simulink model "autonomous_drone"  (R2022a)
settings: Solver=FixedStepAuto  StartTime=0.0  StopTime=inf  FixedStep=sample_time  RelTol=1e-3
PostLoadFcn:
  | addpath("../");
  | load('drone_buses.mat');
InitFcn:
  | rng('shuffle');
StartFcn:
  | rng('shuffle');
model workspace (MAT data in the model file):
  SL_ROS_VariableLengthArrays_MaxSizes.CommonInfo.ArrayTruncateAction = 'EmitWarning'
  SL_ROS_VariableLengthArrays_MaxSizes.MsgTypeMap = containers.Map
  SL_ROS_VariableLengthArrays_MaxSizes.MsgTypeMap.serialization.keys = {'sensor_msgs/Image'}
  SL_ROS_VariableLengthArrays_MaxSizes.MsgTypeMap.serialization.values{1}(1).PropertyName = 'Data'
  SL_ROS_VariableLengthArrays_MaxSizes.MsgTypeMap.serialization.values{1}(1).DataType = 'uint8'
  SL_ROS_VariableLengthArrays_MaxSizes.MsgTypeMap.serialization.values{1}(1).MaxLength = 230400
  SL_ROS_VariableLengthArrays_MaxSizes.MsgTypeMap.serialization.values{1}(2).PropertyName = 'Encoding'
  SL_ROS_VariableLengthArrays_MaxSizes.MsgTypeMap.serialization.values{1}(2).DataType = 'uint8'
  SL_ROS_VariableLengthArrays_MaxSizes.MsgTypeMap.serialization.values{1}(2).MaxLength = 128
  SL_ROS_VariableLengthArrays_MaxSizes.MsgTypeMap.serialization.uniformity = 0
  SL_ROS_VariableLengthArrays_MaxSizes.MsgTypeMap.serialization.keyType = 'char'
  SL_ROS_VariableLengthArrays_MaxSizes.MsgTypeMap.serialization.valueType = 'any'
  cmd_calibration = 0.4
  sample_time = 0.05
undefined symbols (not defined in the file or in its folder): Orientation, Position
libraries: robotlib x11, simulink_extras x4, simulink x2, aerolibanimutils x1, vrlib x1
settings Model: Creator=rcasado  LastModifiedBy=usuario
settings SolverCC: AlgebraicLoopSolver=TrustRegion
settings DataIOCC: ReturnWorkspaceOutputs=off
settings OptimizationCC: EnhancedBackFolding=on  PassReuseOutputArgsAs=Individual arguments  ZeroExternalMemoryAtStartup=off  ZeroInternalMemoryAtStartup=off  MaxStackSize=64  OptimizeBlockOrder=speed  DifferentSizesBufferReuse=on  OptimizationCustomize=off  EfficientTunableParamExpr=on
settings DebuggingCC: ParameterTunabilityLossMsg=error  UnconnectedInputMsg=warning  UnconnectedOutputMsg=warning  UnconnectedLineMsg=warning  BusObjectLabelMismatch=none  PregeneratedLibrarySubsystemCodeDiagnostic=none  SFMachineParentedDataDiag=warning  ArithmeticOperatorsInVariantConditions=warning
settings HardwareCC: ProdBitPerPointer=32  ProdBitPerSizeT=32  ProdBitPerPtrDiffT=32  ProdLargestAtomicFloat=None  ProdIntDivRoundTo=Undefined  ProdEndianess=Unspecified  ProdWordSize=32  ProdHWDeviceType=Generic->Unspecified (assume 32-bit Generic)  UseEmbeddedCoderFeatures=off
settings SFSimCC: SimUseLocalCustomCode=off  MATLABDynamicMemAlloc=off  CustomCodeUndefinedFunction=UseInterfaceOnly
settings RTWCC: SystemTargetFile=ert.tlc  HardwareBoard=Robot Operating System (ROS)  TLCOptions="-aInlineSetEventsForThisBaseRateFcn=TLC_FALSE -aSuppressMultiTaskScheduler=TLC_FALSE  -aRateBasedStepFcn=0"  TemplateMakefile=ert_default_tmf  RTWUseLocalCustomCode=off  Toolchain=Catkin  TargetLang=C++  DLArmComputeVersion=19.05
settings CodeAppCC: ForceParamTrailComments=on  IgnoreCustomStorageClasses=off  OperatorAnnotations=on  SimulinkDataObjDesc=on  SFDataObjDesc=on  InsertBlockDesc=on
settings ERTTargetCC: SupportNonInlinedSFcns=on

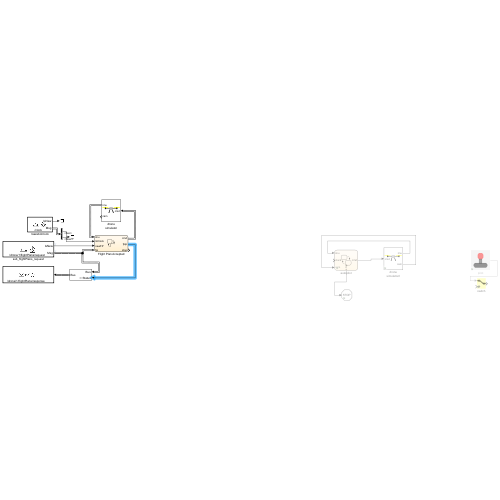
[thumbnail: Simulink's stored preview of the top-level diagram]
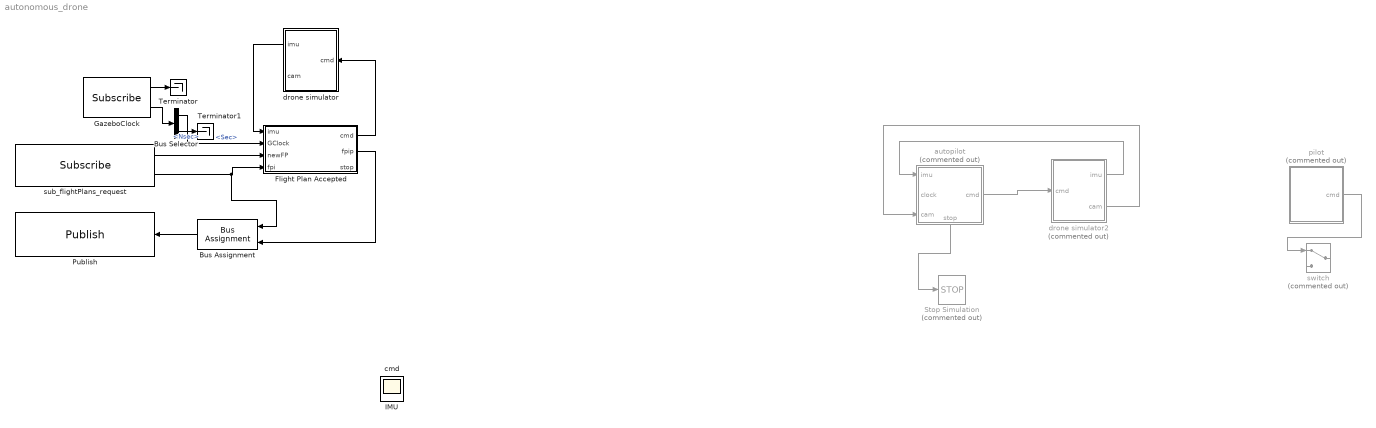
== system autonomous_drone ==
  Bus Assignment : BusAssignment  AssignedSignals=Status
  Bus Selector : BusSelector  OutputSignals=Clock_.Sec,Clock_.Nsec
  Flight Plan Accepted : Stateflow chart  TreatAsAtomicUnit=on
  GazeboClock : robotlib/Subscribe  topicSource=Specify your own  topic=/clock  messageType=rosgraph_msgs/Clock  SampleTime=-1  legacyBusStruct=off  messageQueueLength=1
  Publish : robotlib/Publish  topicSource=Specify your own  topic=/drone/1/flightPlans/response  messageType=siam_main/FlightPlan  legacyBusStruct=off  messageQueueLength=1
  Stop Simulation : Stop  Commented=on
  Terminator : Terminator
  Terminator1 : Terminator
  autopilot : Stateflow chart  Commented=on  TreatAsAtomicUnit=on
      settings: PortSchema="{\"entries\":[{\"content\":{\"sides\":[{\"content\":{\"connectorIds\":[\"In1\",\"In2\",\"In3\"]},\"type\":\"ConnectorPlacement.EquallySpacedRectSide\",\"uuid\":\"89f99594-5326-40e9-9243-02e6688f7e7f\"},{\"content\":{\"connectorIds\":[\"Out1\"],\"side\":\"RIGHT\"},\"type\":\"ConnectorPlacement.EquallySpacedRectSide\",\"uuid\":\"fb6fc64d-4bbc-4560-b28a-cb6226770084\"},{\"content\":{\"connectorIds\":[],\"side\":\"TOP\"},\"type\":\"ConnectorPlacement.EquallySpacedRectSide\",\"uuid\":\"e2b7224a-c622-478e-893e-aabf8760397b\"},{\"content\":{\"connectorIds\":[\"Out2\"],\"side\":\"BOTTOM\"},\"type\":\"ConnectorPlacement.EquallySpacedRectSide\",\"uuid\":\"7db274c0-1c25-455b-8085-b078913bfcbd\"}]},\"type\":\"ConnectorPlacement.EquallySpacedConnector\",\"uuid\":\"69f5fc45-7c88-4079-aa06-728f92b8ad33\"}],\"packageUris\":[\"http://schema.mathworks.com/mf0/Connector/R2020b\"],\"version\":\"1.0\"}"
  drone simulator : Subsystem
      mask Display:
      | patch([50 -50 -50 50], [40 40 -60 -60], [1 1 1])
      | 
      | patch([8 -8 -8 8], [6 6 -6 -6], [0.7 0.7 0.7])
      | 
      | patch([ 8  8  28  28], [2 0 0 2], [0.5 0.5 0.5])
      | patch([-8 -8 -28 -28], [2 0 0 2], [0.5 0.5 0.5])
      | 
      | patch([ 30  46  30  14], [6 5 4 5], [1 1 0])
      | patch([-30 -46 -30 -14], [6 5 4 5], [1 1 0])
      | 
      | patch([ 28  28  32  32], [4 -2 -2 4], [0 0 0])
      | patch([-28 -28 -32 -32], [4 -2 -2 4], [0 0 0])
      | 
      | patch([ 8  12  11  7], [-6 -18 -18 -6], [0 0 0])
      | patch([-8 -12 -11 -7], [-6 -18 -18 -6], [0 0 0])
  drone simulator2 : Subsystem  Commented=on
      mask Display:
      | patch([50 -50 -50 50], [40 40 -60 -60], [1 1 1])
      | 
      | patch([8 -8 -8 8], [6 6 -6 -6], [0.7 0.7 0.7])
      | 
      | patch([ 8  8  28  28], [2 0 0 2], [0.5 0.5 0.5])
      | patch([-8 -8 -28 -28], [2 0 0 2], [0.5 0.5 0.5])
      | 
      | patch([ 30  46  30  14], [6 5 4 5], [1 1 0])
      | patch([-30 -46 -30 -14], [6 5 4 5], [1 1 0])
      | 
      | patch([ 28  28  32  32], [4 -2 -2 4], [0 0 0])
      | patch([-28 -28 -32 -32], [4 -2 -2 4], [0 0 0])
      | 
      | patch([ 8  12  11  7], [-6 -18 -18 -6], [0 0 0])
      | patch([-8 -12 -11 -7], [-6 -18 -18 -6], [0 0 0])
  pilot : Subsystem  Commented=on
      mask Display:
      | patch([12 -2 -2 12], [12 12 -2 -2], [0.9 0.9 0.9])
      | 
      | % bola roja
      | patch([4 6 7 7 6 4 3 3], [6 6 7 9 10 10 9 7], [1 0 0])
      | 
      | % palo gris
      | patch([4 6 6 4], [3 3 6 6], [0.2 0.2 0.2])
      | 
      | % base negra
      | patch([1 9 10 10 9 1 0 0], [0 0 1 2 3 3 2 1], [0 0 0])
  sub_flightPlans_request : robotlib/Subscribe  topicSource=Specify your own  topic=/drone/1/flightPlans/request  messageType=siam_main/FlightPlan  SampleTime=0.05  legacyBusStruct=off  messageQueueLength=1
  switch : ManualSwitch  Commented=on
  IMU : Scope
  cmd : Scope
  wires:
  autopilot/1(cmd) -> drone simulator2/1(cmd)
  drone simulator2/1(imu) -> autopilot/1(imu)
  drone simulator2/2(cam) -> autopilot/3(cam)
  pilot/1(cmd) -> switch/1
  autopilot/2(stop) -> Stop Simulation/1
  GazeboClock/1 -> Terminator/1
  GazeboClock/2 -> Bus Selector/1
  Bus Selector/2 -> Terminator1/1  "<Nsec>"
  sub_flightPlans_request/1 -> Flight Plan Accepted/3(newFP)
  sub_flightPlans_request/2 -> Bus Assignment/1, Flight Plan Accepted/4(fpi)
  Flight Plan Accepted/1(cmd) -> drone simulator/1(cmd)
  drone simulator/1(imu) -> Flight Plan Accepted/1(imu)
  Bus Selector/1 -> Flight Plan Accepted/2(GClock)  "<Sec>"
  Bus Assignment/1 -> Publish/1
  Flight Plan Accepted/2(fpip) -> Bus Assignment/2

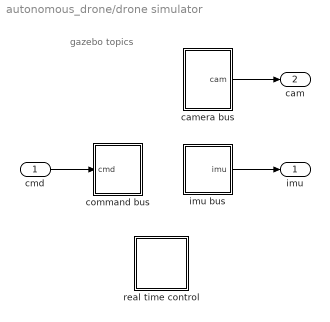
== system autonomous_drone/drone simulator ==
  note: gazebo
      | topics
  cmd : Inport
  camera bus : Subsystem
  command bus : Subsystem
  imu bus : Subsystem
  real time control : Subsystem
      mask Display: disp('realtime\ncontrol')
  imu : Outport  VectorParamsAs1DForOutWhenUnconnected=off
  cam : Outport  Port=2  VectorParamsAs1DForOutWhenUnconnected=off
  wires:
  camera bus/1(cam) -> cam/1
  cmd/1 -> command bus/1(cmd)
  imu bus/1(imu) -> imu/1

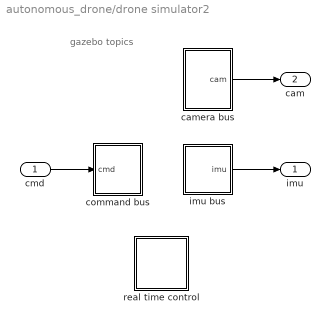
== system autonomous_drone/drone simulator2 ==
  note: gazebo
      | topics
  cmd : Inport
  camera bus : Subsystem
  command bus : Subsystem
  imu bus : Subsystem
  real time control : Subsystem
      mask Display: disp('realtime\ncontrol')
  imu : Outport  VectorParamsAs1DForOutWhenUnconnected=off
  cam : Outport  Port=2  VectorParamsAs1DForOutWhenUnconnected=off
  wires:
  imu bus/1(imu) -> imu/1
  cmd/1 -> command bus/1(cmd)
  camera bus/1(cam) -> cam/1

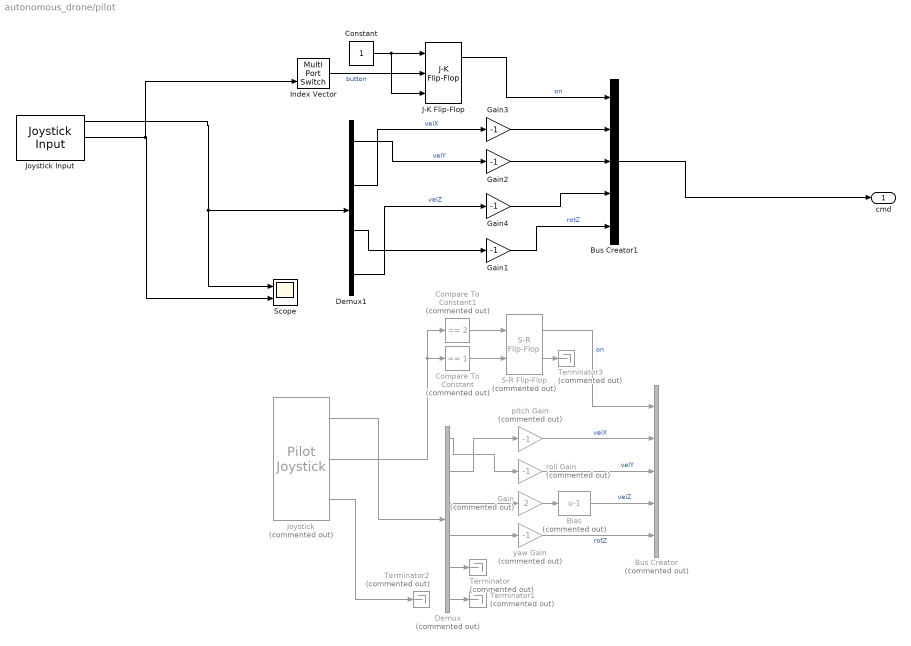
== system autonomous_drone/pilot ==
  Bias : Bias  Commented=on  Bias=-1  SaturateOnIntegerOverflow=off
  Bus Creator : BusCreator  Commented=on  Inputs=5  OutDataTypeStr=Bus: bus_command  NonVirtualBus=on
      settings: InheritFromInputs=off
  Bus Creator1 : BusCreator  Inputs=5  OutDataTypeStr=Bus: bus_command  NonVirtualBus=on
      settings: InheritFromInputs=off
  Compare To Constant : simulink/Logic and Bit Operations/Compare To Constant  Commented=on  relop===  const=1  OutDataTypeStr=boolean
  Compare To Constant1 : simulink/Logic and Bit Operations/Compare To Constant  Commented=on  relop===  const=2  OutDataTypeStr=boolean
  Constant : Constant  OutDataTypeStr=boolean
  Demux : Demux  Commented=on  Outputs=6
  Demux1 : Demux
  Gain : Gain  Commented=on  Gain=2
  Gain{1..4} (4 alike) : Gain  Gain=-1
  Index Vector : MultiPortSwitch  DataPortOrder=Zero-based contiguous  Inputs=1  zeroidx=on  SaturateOnIntegerOverflow=off  InputSameDT=off
  J-K Flip-Flop : simulink_extras/Flip Flops/J-K Flip-Flop  initial_condition=0
  Joystick : aerolibanimutils/Pilot Joystick  Commented=on  JoystickID=Joystick1  OutputConfiguration=AllOutputs  SampleTime=sample_time
  Joystick Input : vrlib/Joystick Input  joyid=1  adjustports=on  forcefeed=off
  S-R Flip-Flop : simulink_extras/Flip Flops/S-R Flip-Flop  Commented=on  initial_condition=0
  Scope : Scope  NumInputPorts=2
  Terminator{,1..3} (4 alike) : Terminator  Commented=on
  pitch Gain : Gain  Commented=on  Gain=-1
  roll Gain : Gain  Commented=on  Gain=-1
  yaw Gain : Gain  Commented=on  Gain=-1
  cmd : Outport  VectorParamsAs1DForOutWhenUnconnected=off
  wires:
  Demux/4 -> yaw Gain/1
  Demux/3 -> Gain/1
  Demux/1 -> roll Gain/1
  Demux/2 -> pitch Gain/1
  Gain/1 -> Bias/1
  Bias/1 -> Bus Creator/4  "velZ"
  yaw Gain/1 -> Bus Creator/5  "rotZ"
  pitch Gain/1 -> Bus Creator/2  "velX"
  roll Gain/1 -> Bus Creator/3  "velY"
  S-R Flip-Flop/1 -> Bus Creator/1  "on"
  Joystick/1 -> Demux/1
  Demux/6 -> Terminator1/1
  Demux/5 -> Terminator/1
  Joystick/2 -> Compare To Constant1/1, Compare To Constant/1
  Joystick/3 -> Terminator2/1
  Compare To Constant/1 -> S-R Flip-Flop/2
  Compare To Constant1/1 -> S-R Flip-Flop/1
  S-R Flip-Flop/2 -> Terminator3/1
  Demux1/1 -> Gain2/1  "velY"
  Demux1/2 -> Gain3/1  "velX"
  Demux1/4 -> Gain4/1  "velZ"
  J-K Flip-Flop/1 -> Bus Creator1/1  "on"
  Bus Creator1/1 -> cmd/1
  Demux1/3 -> Gain1/1
  Gain1/1 -> Bus Creator1/5  "rotZ"
  Gain2/1 -> Bus Creator1/3
  Index Vector/1 -> J-K Flip-Flop/2  "button"
  Constant/1 -> J-K Flip-Flop/3, J-K Flip-Flop/1
  Gain3/1 -> Bus Creator1/2
  Gain4/1 -> Bus Creator1/4
  Joystick Input/1 -> Demux1/1, Scope/1
  Joystick Input/2 -> Index Vector/2, Scope/2

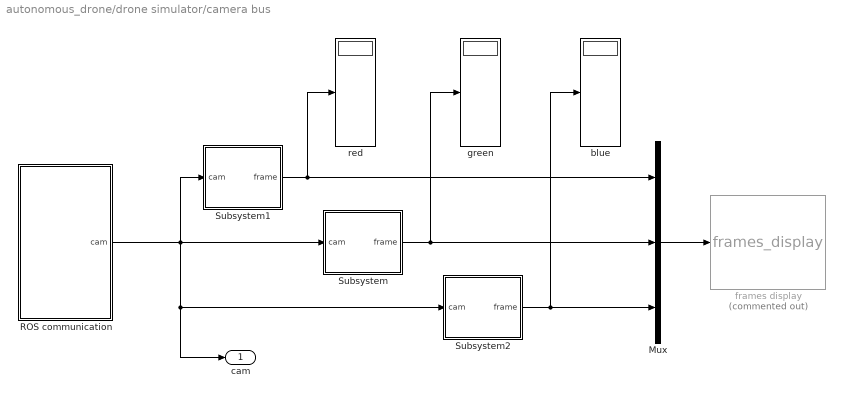
== system autonomous_drone/drone simulator/camera bus ==
  Mux : Mux  Inputs=3
  ROS communication : Subsystem
  Subsystem : Subsystem
  Subsystem1 : Subsystem
  Subsystem2 : Subsystem
  blue : Display
  frames display : MATLABFcn  Commented=on  StartFcn=|  MATLABFcn=frames_display  OutputDimensions=0  Output1D=off
      | clear functions;
      | clc;
      mask Display:
      | patch([80 100 100 80], [60 60 80 80],[1 0 0])
      | 
      | patch([60 75 75 60], [20 20 30 30],[0 1 0])
      | 
      | patch([20 40 40 20], [40 40 50 50],[0 0 1])
  green : Display
  red : Display
  cam : Outport  VectorParamsAs1DForOutWhenUnconnected=off
  wires:
  Subsystem1/1(frame) -> Mux/1, red/1
  ROS communication/1(cam) -> Subsystem/1(cam), Subsystem1/1(cam), Subsystem2/1(cam), cam/1
  Subsystem2/1(frame) -> Mux/3, blue/1
  Subsystem/1(frame) -> Mux/2, green/1
  Mux/1 -> frames display/1

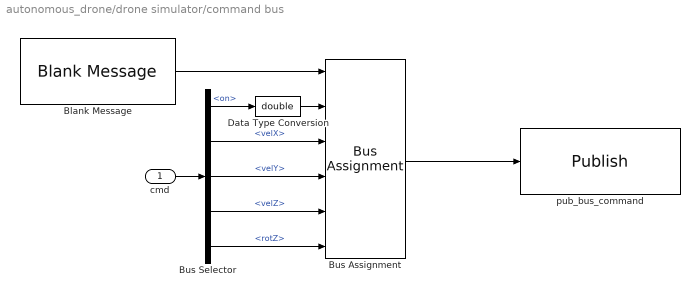
== system autonomous_drone/drone simulator/command bus ==
  cmd : Inport
  Blank Message : robotlib/Blank Message  messageClass=Message  entityType=geometry_msgs/Pose  messageType=geometry_msgs/Pose  SampleTime=sample_time  legacyBusStruct=off
  Bus Assignment : BusAssignment  AssignedSignals=Position.X,Orientation.X,Orientation.Y,Orientation.Z,Orientation.W
  Bus Selector : BusSelector  OutputSignals=on,velX,velY,velZ,rotZ
  Data Type Conversion : DataTypeConversion  OutDataTypeStr=double  SaturateOnIntegerOverflow=off  RndMeth=Floor
  pub_bus_command : robotlib/Publish  topicSource=Specify your own  topic=/drone/1/bus_command  messageType=geometry_msgs/Pose  legacyBusStruct=off  messageQueueLength=105
  wires:
  Data Type Conversion/1 -> Bus Assignment/2
  Bus Selector/5 -> Bus Assignment/6  "<rotZ>"
  Bus Selector/1 -> Data Type Conversion/1  "<on>"
  Bus Selector/2 -> Bus Assignment/3  "<velX>"
  Bus Selector/3 -> Bus Assignment/4  "<velY>"
  Bus Selector/4 -> Bus Assignment/5  "<velZ>"
  Blank Message/1 -> Bus Assignment/1
  cmd/1 -> Bus Selector/1
  Bus Assignment/1 -> pub_bus_command/1

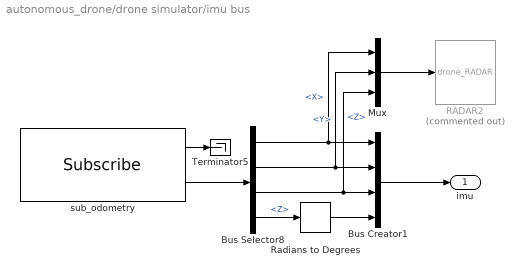
== system autonomous_drone/drone simulator/imu bus ==
  Bus Creator1 : BusCreator  Inputs=4  OutDataTypeStr=Bus: bus_IMU  NonVirtualBus=on
      settings: InheritFromInputs=off
  Bus Selector8 : BusSelector  DialogController=Simulink.DDGSource_BusSelector  OutputSignals=Pose.Position.X,Pose.Position.Y,Pose.Position.Z,Pose.Orientation.Z
  Mux : Mux  Inputs=3
  RADAR2 : MATLABFcn  Commented=on  StartFcn=|  MATLABFcn=drone_RADAR  OutputDimensions=0  Output1D=off
      | clear functions;
      | clc;
      mask Display:
      | plot([00 10], [05 05])
      | plot([05 05], [00 10])
      | 
      | plot([01 09 09 01 01], [01 01 09 09 01])
      | plot([03 07 07 03 03], [03 03 07 07 03])
  Radians to Degrees : simulink_extras/Transformations/Radians to Degrees
  Terminator5 : Terminator
  sub_odometry : robotlib/Subscribe  topicSource=Specify your own  topic=/drone/1/odometry  messageType=gazebo_msgs/ModelState  SampleTime=sample_time  legacyBusStruct=off  messageQueueLength=51
  imu : Outport  VectorParamsAs1DForOutWhenUnconnected=off
  wires:
  Mux/1 -> RADAR2/1
  sub_odometry/2 -> Bus Selector8/1
  Radians to Degrees/1 -> Bus Creator1/4
  Bus Creator1/1 -> imu/1
  Bus Selector8/1 -> Mux/1, Bus Creator1/1  "<X>"
  Bus Selector8/3 -> Mux/3, Bus Creator1/3  "<Z>"
  Bus Selector8/2 -> Mux/2, Bus Creator1/2  "<Y>"
  Bus Selector8/4 -> Radians to Degrees/1  "<Z>"
  sub_odometry/1 -> Terminator5/1

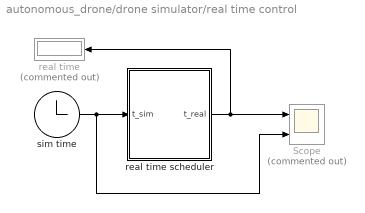
== system autonomous_drone/drone simulator/real time control ==
  Scope : Scope  Commented=on  NumInputPorts=2
  real time : Display  Commented=on
      settings: Format=bank
  real time scheduler : MATLAB Function  TreatAsAtomicUnit=on
  sim time : Clock
  wires:
  sim time/1 -> Scope/2, real time scheduler/1(t_sim)
  real time scheduler/1(t_real) -> Scope/1, real time/1

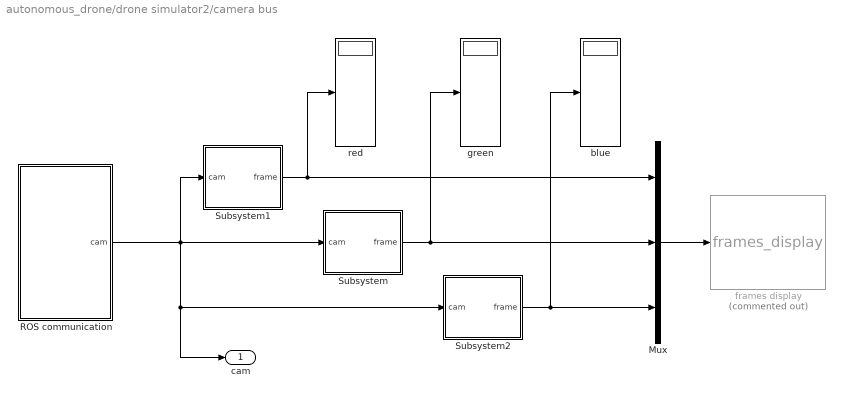
== system autonomous_drone/drone simulator2/camera bus ==
  Mux : Mux  Inputs=3
  ROS communication : Subsystem
  Subsystem : Subsystem
  Subsystem1 : Subsystem
  Subsystem2 : Subsystem
  blue : Display
  frames display : MATLABFcn  Commented=on  StartFcn=|  MATLABFcn=frames_display  OutputDimensions=0  Output1D=off
      | clear functions;
      | clc;
      mask Display:
      | patch([80 100 100 80], [60 60 80 80],[1 0 0])
      | 
      | patch([60 75 75 60], [20 20 30 30],[0 1 0])
      | 
      | patch([20 40 40 20], [40 40 50 50],[0 0 1])
  green : Display
  red : Display
  cam : Outport  VectorParamsAs1DForOutWhenUnconnected=off
  wires:
  Mux/1 -> frames display/1
  Subsystem/1(frame) -> green/1, Mux/2
  Subsystem2/1(frame) -> blue/1, Mux/3
  ROS communication/1(cam) -> cam/1, Subsystem2/1(cam), Subsystem1/1(cam), Subsystem/1(cam)
  Subsystem1/1(frame) -> red/1, Mux/1

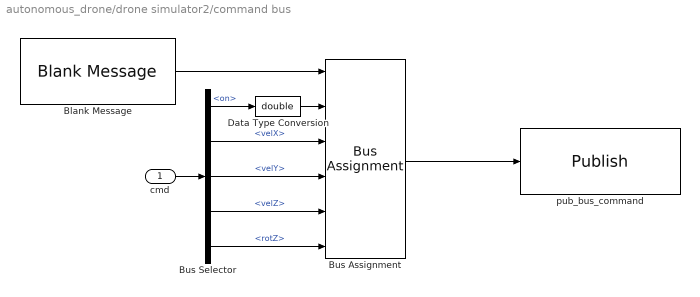
== system autonomous_drone/drone simulator2/command bus ==
  cmd : Inport
  Blank Message : robotlib/Blank Message  messageClass=Message  entityType=geometry_msgs/Pose  messageType=geometry_msgs/Pose  SampleTime=sample_time  legacyBusStruct=off
  Bus Assignment : BusAssignment  AssignedSignals=Position.X,Orientation.X,Orientation.Y,Orientation.Z,Orientation.W
  Bus Selector : BusSelector  OutputSignals=on,velX,velY,velZ,rotZ
  Data Type Conversion : DataTypeConversion  OutDataTypeStr=double  SaturateOnIntegerOverflow=off  RndMeth=Floor
  pub_bus_command : robotlib/Publish  topicSource=Specify your own  topic=/drone/1/bus_command  messageType=geometry_msgs/Pose  legacyBusStruct=off  messageQueueLength=105
  wires:
  Bus Assignment/1 -> pub_bus_command/1
  cmd/1 -> Bus Selector/1
  Blank Message/1 -> Bus Assignment/1
  Bus Selector/4 -> Bus Assignment/5  "<velZ>"
  Bus Selector/3 -> Bus Assignment/4  "<velY>"
  Bus Selector/2 -> Bus Assignment/3  "<velX>"
  Bus Selector/1 -> Data Type Conversion/1  "<on>"
  Bus Selector/5 -> Bus Assignment/6  "<rotZ>"
  Data Type Conversion/1 -> Bus Assignment/2

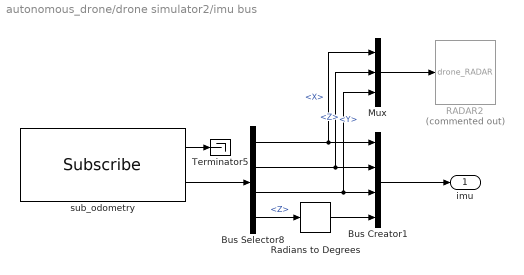
== system autonomous_drone/drone simulator2/imu bus ==
  Bus Creator1 : BusCreator  Inputs=4  OutDataTypeStr=Bus: bus_IMU  NonVirtualBus=on
      settings: InheritFromInputs=off
  Bus Selector8 : BusSelector  DialogController=Simulink.DDGSource_BusSelector  OutputSignals=Pose.Position.X,Pose.Position.Y,Pose.Position.Z,Pose.Orientation.Z
  Mux : Mux  Inputs=3
  RADAR2 : MATLABFcn  Commented=on  StartFcn=|  MATLABFcn=drone_RADAR  OutputDimensions=0  Output1D=off
      | clear functions;
      | clc;
      mask Display:
      | plot([00 10], [05 05])
      | plot([05 05], [00 10])
      | 
      | plot([01 09 09 01 01], [01 01 09 09 01])
      | plot([03 07 07 03 03], [03 03 07 07 03])
  Radians to Degrees : simulink_extras/Transformations/Radians to Degrees
  Terminator5 : Terminator
  sub_odometry : robotlib/Subscribe  topicSource=Specify your own  topic=/drone/1/odometry  messageType=gazebo_msgs/ModelState  SampleTime=sample_time  legacyBusStruct=off  messageQueueLength=51
  imu : Outport  VectorParamsAs1DForOutWhenUnconnected=off
  wires:
  sub_odometry/1 -> Terminator5/1
  Bus Selector8/4 -> Radians to Degrees/1  "<Z>"
  Bus Selector8/2 -> Bus Creator1/2, Mux/2  "<Y>"
  Bus Selector8/3 -> Bus Creator1/3, Mux/3  "<Z>"
  Bus Selector8/1 -> Bus Creator1/1, Mux/1  "<X>"
  Bus Creator1/1 -> imu/1
  Radians to Degrees/1 -> Bus Creator1/4
  sub_odometry/2 -> Bus Selector8/1
  Mux/1 -> RADAR2/1

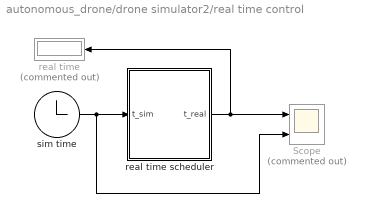
== system autonomous_drone/drone simulator2/real time control ==
  Scope : Scope  Commented=on  NumInputPorts=2
  real time : Display  Commented=on
      settings: Format=bank
  real time scheduler : MATLAB Function  TreatAsAtomicUnit=on
  sim time : Clock
  wires:
  real time scheduler/1(t_real) -> real time/1, Scope/1
  sim time/1 -> real time scheduler/1(t_sim), Scope/2

== system autonomous_drone/drone simulator/camera bus/ROS communication ==
  Terminator2 : Terminator
  sub_camera : robotlib/Subscribe  topicSource=Specify your own  topic=/drone/1/onboard_camera/image_raw  messageType=sensor_msgs/Image  SampleTime=sample_time  legacyBusStruct=off  messageQueueLength=51
  vision : MATLAB Function  TreatAsAtomicUnit=on
  cam : Outport  VectorParamsAs1DForOutWhenUnconnected=off
  wires:
  sub_camera/1 -> Terminator2/1
  sub_camera/2 -> vision/1(message)
  vision/1(cam) -> cam/1

== system autonomous_drone/drone simulator/camera bus/Subsystem ==
  cam : Inport
  Bus Selector1 : BusSelector  OutputSignals=green.n,green.s,green.e,green.w,green.d,green.a
  Mux1 : Mux  Inputs=6
  frame : Outport  VectorParamsAs1DForOutWhenUnconnected=off
  wires:
  Bus Selector1/2 -> Mux1/2  "<s>"
  Mux1/1 -> frame/1
  Bus Selector1/1 -> Mux1/1  "<n>"
  cam/1 -> Bus Selector1/1
  Bus Selector1/4 -> Mux1/4  "<w>"
  Bus Selector1/5 -> Mux1/5  "<d>"
  Bus Selector1/6 -> Mux1/6  "<a>"
  Bus Selector1/3 -> Mux1/3  "<e>"

== system autonomous_drone/drone simulator/camera bus/Subsystem1 ==
  cam : Inport
  Bus Selector1 : BusSelector  OutputSignals=red.n,red.s,red.e,red.w,red.d,red.a
  Mux1 : Mux  Inputs=6
  frame : Outport  VectorParamsAs1DForOutWhenUnconnected=off
  wires:
  Bus Selector1/2 -> Mux1/2  "<s>"
  Mux1/1 -> frame/1
  Bus Selector1/1 -> Mux1/1  "<n>"
  cam/1 -> Bus Selector1/1
  Bus Selector1/4 -> Mux1/4  "<w>"
  Bus Selector1/5 -> Mux1/5  "<d>"
  Bus Selector1/6 -> Mux1/6  "<a>"
  Bus Selector1/3 -> Mux1/3  "<e>"

== system autonomous_drone/drone simulator/camera bus/Subsystem2 ==
  cam : Inport
  Bus Selector1 : BusSelector  OutputSignals=blue.n,blue.s,blue.e,blue.w,blue.d,blue.a
  Mux1 : Mux  Inputs=6
  frame : Outport  VectorParamsAs1DForOutWhenUnconnected=off
  wires:
  Bus Selector1/2 -> Mux1/2  "<s>"
  Mux1/1 -> frame/1
  Bus Selector1/1 -> Mux1/1  "<n>"
  cam/1 -> Bus Selector1/1
  Bus Selector1/4 -> Mux1/4  "<w>"
  Bus Selector1/5 -> Mux1/5  "<d>"
  Bus Selector1/6 -> Mux1/6  "<a>"
  Bus Selector1/3 -> Mux1/3  "<e>"

== system autonomous_drone/drone simulator2/camera bus/ROS communication ==
  Terminator2 : Terminator
  sub_camera : robotlib/Subscribe  topicSource=Specify your own  topic=/drone/1/onboard_camera/image_raw  messageType=sensor_msgs/Image  SampleTime=sample_time  legacyBusStruct=off  messageQueueLength=51
  vision : MATLAB Function  TreatAsAtomicUnit=on
  cam : Outport  VectorParamsAs1DForOutWhenUnconnected=off
  wires:
  vision/1(cam) -> cam/1
  sub_camera/2 -> vision/1(message)
  sub_camera/1 -> Terminator2/1

== system autonomous_drone/drone simulator2/camera bus/Subsystem ==
  cam : Inport
  Bus Selector1 : BusSelector  OutputSignals=green.n,green.s,green.e,green.w,green.d,green.a
  Mux1 : Mux  Inputs=6
  frame : Outport  VectorParamsAs1DForOutWhenUnconnected=off
  wires:
  Bus Selector1/3 -> Mux1/3  "<e>"
  Bus Selector1/6 -> Mux1/6  "<a>"
  Bus Selector1/5 -> Mux1/5  "<d>"
  Bus Selector1/4 -> Mux1/4  "<w>"
  cam/1 -> Bus Selector1/1
  Bus Selector1/1 -> Mux1/1  "<n>"
  Mux1/1 -> frame/1
  Bus Selector1/2 -> Mux1/2  "<s>"

== system autonomous_drone/drone simulator2/camera bus/Subsystem1 ==
  cam : Inport
  Bus Selector1 : BusSelector  OutputSignals=red.n,red.s,red.e,red.w,red.d,red.a
  Mux1 : Mux  Inputs=6
  frame : Outport  VectorParamsAs1DForOutWhenUnconnected=off
  wires:
  Bus Selector1/3 -> Mux1/3  "<e>"
  Bus Selector1/6 -> Mux1/6  "<a>"
  Bus Selector1/5 -> Mux1/5  "<d>"
  Bus Selector1/4 -> Mux1/4  "<w>"
  cam/1 -> Bus Selector1/1
  Bus Selector1/1 -> Mux1/1  "<n>"
  Mux1/1 -> frame/1
  Bus Selector1/2 -> Mux1/2  "<s>"

== system autonomous_drone/drone simulator2/camera bus/Subsystem2 ==
  cam : Inport
  Bus Selector1 : BusSelector  OutputSignals=blue.n,blue.s,blue.e,blue.w,blue.d,blue.a
  Mux1 : Mux  Inputs=6
  frame : Outport  VectorParamsAs1DForOutWhenUnconnected=off
  wires:
  Bus Selector1/3 -> Mux1/3  "<e>"
  Bus Selector1/6 -> Mux1/6  "<a>"
  Bus Selector1/5 -> Mux1/5  "<d>"
  Bus Selector1/4 -> Mux1/4  "<w>"
  cam/1 -> Bus Selector1/1
  Bus Selector1/1 -> Mux1/1  "<n>"
  Mux1/1 -> frame/1
  Bus Selector1/2 -> Mux1/2  "<s>"

== matlab function autonomous_drone/drone simulator2/camera bus/ROS communication/vision ==
  data: message input; cam output Bus: bus_camera
function cam = fcn(message)

% leemos la imagen
width  = message.Width;
height = message.Height;
img    = message.Data;

% establecemos los valores umbrales de deteccion de color
th1 = 50;         % umbral entre color primario y secundarios
th2 = 20;         % umbral entre colores secundarios

% marco rojo
frame_red.d = +inf;        % distancia estimada
frame_red.a = +inf;        % angulo de entrada estimado
frame_red.n = +inf;        % lado norte
frame_red.s = -inf;        % lado sur
frame_red.e = -inf;        % lado este
frame_red.w = +inf;        % lado oeste

% marco verde
frame_green = frame_red;      
% marco azul
frame_blue = frame_red; 


% deteccion de rectangulos conteniendo los pixeles de cada marco
i = 1;
for row = 1:height %240
for col = 1:width  %320

    r = double(img(i));  i=i+1;
    g = double(img(i));  i=i+1;
    b = double(img(i));  i=i+1;
    
    if(abs(g-b) < th2) && ((r-g) > th1)        %rojo
        if(frame_red.n > row) 
           frame_red.n = double(row);
        end
        if(frame_red.s < row) 
           frame_red.s = double(row);
        end
        if(frame_red.e < col) 
           frame_red.e = double(col);
        end
        if(frame_red.w > col) 
           frame_red.w = double(col);
        end
    elseif(abs(b-r) < th2) && ((g-b) > th1)    %verde
        if(frame_green.n > row) 
           frame_green.n = double(row);
        end
        if(frame_green.s < row) 
           frame_green.s = double(row);
        end
        if(frame_green.e < col) 
           frame_green.e = double(col);
        end
        if(frame_green.w > col) 
           frame_green.w = double(col);
        end
    elseif(abs(r-g) < th2) && ((b-r) > th1)    %azul
        if(frame_blue.n > row) 
           frame_blue.n = double(row);
        end
        if(frame_blue.s < row) 
           frame_blue.s = double(row);
        end
        if(frame_blue.e < col) 
           frame_blue.e = double(col);
        end
        if(frame_blue.w > col) 
           frame_blue.w = double(col);
        end
    end
    
end
end

% Cambio del sistema de coordenadas de la imagen
frame_red.n   = 120 - frame_red.n;
frame_red.s   = 120 - frame_red.s;
frame_red.e   = frame_red.e - 161;
frame_red.w   = frame_red.w - 161;

frame_green.n = 120 - frame_green.n;
frame_green.s = 120 - frame_green.s;
frame_green.e = frame_green.e - 161;
frame_green.w = frame_green.w - 161;

frame_blue.n  = 120 - frame_blue.n;
frame_blue.s  = 120 - frame_blue.s;
frame_blue.e  = frame_blue.e - 161;
frame_blue.w  = frame_blue.w - 161;


%% Analisis de posicion (distancia, y angulos de deriva/entrada)

d2 = 160^2;    % 160^2 pixeles
L  = 0.23;       % alto de marco
A  = 0.43;       % ancho del marco

if frame_red.n > -inf && frame_red.n < 119 && frame_red.s > -120
    l = frame_red.n - frame_red.s;
    h = frame_red.s + l/2;
    frame_red.d = L/l * sqrt(d2 + h^2);
    ap = frame_red.e - frame_red.w;
    a = max(A/L * l,ap);
    frame_red.a = acosd(ap/a);
end

if frame_green.n > -inf && frame_green.n < 119 && frame_green.s > -120
    l = frame_green.n - frame_green.s;
    h = frame_green.s + l/2;
    frame_green.d = L/l * sqrt(d2 + h^2);
    ap = frame_green.e - frame_green.w;
    a = max(A/L * l,ap);
    frame_green.a = acosd(ap/a);
end

if frame_blue.n > -inf && frame_blue.n < 119 && frame_blue.s > -120
    l = frame_blue.n - frame_blue.s;
    h = frame_blue.s + l/2;
    frame_blue.d = L/l * sqrt(d2 + h^2);
    ap = frame_blue.e - frame_blue.w;
    a = max(A/L * l,ap);
    frame_blue.a = acosd(ap/a);
end




%% Enviamos informacion por el topic
cam.red = frame_red;
cam.green = frame_green;
cam.blue = frame_blue;

== matlab function autonomous_drone/drone simulator2/real time control/real time scheduler ==
  data: t_sim input; t_real output
function t_real = fcn(t_sim)
%#codegen

coder.extrinsic('tic');
coder.extrinsic('toc');

persistent t0;
if isempty(t0)
    t0 = tic;
    t_real = 0;
end

t_real = toc(t0);

t_dif = t_sim - t_real;
if t_dif > 0
%    disp(t_dif)
    pause(t_dif);
end

t_real = toc(t0);
%disp(t_real)

== stateflow chart autonomous_drone/autopilot ==
  settings: updateMethod=DISCRETE  sampleTime=sample_time  executeAtInitialization=1
  state Navigation
    state Navigation
      entry:
      disp("Navigating until waypoint " + waypointIndex);
    state Start
      entry:
      Hover();
      waypointIndex = 1;
    state WaypointReached
      entry:
      waypointIndex = waypointIndex + 1;
    state End
    (default) -> Navigation.Start
    Navigation.Start -> Navigation.Navigation
    WaypointReached -> Navigation.Navigation [order 1] : [NextWaypoint(waypointIndex,route) == 1]
    Navigation.Navigation -> WaypointReached : [Fly2(route(waypointIndex,1),route(waypointIndex,2),route(waypointIndex,3)) < 0.5]
    WaypointReached -> Navigation.End [order 2] : [NextWaypoint(waypointIndex,route) == 0]
  state TakeOff
    state End
    state SetBase
      entry:
      posInit = [imu.posX, imu.posY, imu.posZ];
    state Start
      entry:
      Hover();
      route = [
      [-4, -4, 2],
      [-4, 4, 3],
      [4,4,2],
      [4,-4, 1]
      ]
    SetBase -> TakeOff.End : [Fly2(posInit(1), posInit(2), 1)<0.1]
    TakeOff.Start -> SetBase
    (default) -> TakeOff.Start
  state Landing
    state Go2Base
    state Stop
      entry:
      cmd.on = false;
    state StopSimul
      entry:
      stop = 1;
    (default) -> Go2Base
    Go2Base -> Stop : [Fly2(posInit(1), posInit(2), 0.6)<0.05]
    Stop -> StopSimul : after(3,sec)
  state WaitingInit
  TakeOff.End -> Navigation
  WaitingInit -> TakeOff : [clock < 10]
  (default) -> WaitingInit
  Navigation.End -> Landing
  data: moreWaypoint function_output; index function_input; route function_input; X function_input; d3D function_output; Y function_input; Z function_input; id function_input; imu input Bus: bus_IMU size=1; clock input; cmd output Bus: bus_command size=1; cam input Bus: bus_camera size=1; posInit local; initA local; route local; waypointIndex local int16; stop output double size=1 =0
  function moreWaypoint = NextWaypoint(index, route):
    | function moreWaypoint = NextWaypoint(index, route)
    |     if length(route) == index
    |         moreWaypoint = 0;
    |     else
    |         moreWaypoint = 1;
    |     end
    | end
  function d3D = Fly2(X,Y,Z):
    | function d3D = Fly2(X,Y,Z)
    | 
    | % target distance decomposed into earth axes
    | %vector between the commanded position and the drone position
    | dxe = X - imu.posX;
    | dye = Y - imu.posY;
    | dze = Z - imu.posZ;
    | 
    | % target distance
    | % vector3D modulus
    | d3D = norm([dxe;dye;dze]);
    | 
    | % target distance on the plane
    | %vector2D modulus
    | d2D = norm([dxe;dye]);
    | 
    | % angle between drone heading and target
    | %As commanded velocity is relative to drone heading, 
    | %difference between heading and target must be computed in order to compute
    | %the correct drone displacement
    | bearing = atan2d(dye, dxe) - imu.rumbo;
    | 
    | % target distance decomposed into drone body axes
    | %distance transformed to drone taking into account drone heading
    | dx = d2D * cosd(bearing);
    | dy = d2D * sind(bearing);
    | dz = dze;
    | 
    | % velocity obtained from distance
    | % speed softened (50%)
    | vel = [dx;dy;dz]/2;
    | % speed normalization
    | if norm(vel) > 1 
    |     vel = vel / norm(vel);
    | end
    | 
    | %Speeed commanded
    | cmd.velX = vel(1);
    | cmd.velY = vel(2);
    | cmd.velZ = vel(3);
  function Hover:
    | function Hover
    | 
    | %Keep the drone in the air without displacement
    | cmd.on   = true;
    | cmd.velX = 0;
    | cmd.velY = 0;
    | cmd.velZ = 0;
    | cmd.rotZ = 0;
  function Look2Frame(id):
    | function Look2Frame(id)
    | 
    | %Selection of the frame to look at
    | switch id
    |     case 'red'
    |         fr = cam.red;
    |     case 'green'
    |         fr = cam.green;
    |     case 'blue'
    |         fr = cam.blue;
    | end
    | 
    | %Get the displacement necesary to be in the middle of the frame
    | if (fr.d ~= inf)
    |     HorCenter = (fr.e + fr.w)/2;
    |     cmd.rotZ  = - HorCenter/80;
    |     VerCenter = (fr.n + fr.s)/2;
    |     cmd.velZ  = VerCenter/120;
    | end

== stateflow chart autonomous_drone/Flight Plan Accepted ==
  state FlightPlanReceived
    entry:
    fpip = 1;
    fp = fpi;
  state WaitingFlightPlan
    entry:
    fpip = 0;
  state TakeOff
    state End
    state SetBase
      entry:
      %posInit = [fp.Orig.X, fp.Orig.Y, fp.Orig.Z];
    state Start
      entry:
      Hover();
      route = fp.Route;
      routeL = fp.Route_SL_Info.CurrentLength;
    SetBase -> TakeOff.End : [Fly2(fp.Orig.X, fp.Orig.Y, fp.Orig.Z)<0.1]
    TakeOff.Start -> SetBase
    (default) -> TakeOff.Start
  state Landing
    state Go2Base
    state Stop
      entry:
      cmd.on = false;
    state StopSimul
      entry:
      fpip = 2;
      stop = 1;
    (default) -> Go2Base
    Go2Base -> Stop : [Fly2(fp.Dest.X, fp.Dest.Y, fp.Dest.Z)<0.1]
    Stop -> StopSimul : after(3,sec)
  state Navigation
    state Navigation
      entry:
      disp("Navigating until waypoint " + waypointIndex);
    state Start
      entry:
      Hover();
      waypointIndex = 1;
    state WaypointReached
      entry:
      waypointIndex = waypointIndex + 1;
    state End
    WaypointReached -> Navigation.Navigation [order 1] : [NextWaypoint(waypointIndex,route, routeL) == 1]
    (default) -> Navigation.Start
    Navigation.Start -> Navigation.Navigation
    Navigation.Navigation -> WaypointReached : [Fly2(route(waypointIndex).X,route(waypointIndex).Y,route(waypointIndex).Z) < 0.5]
    WaypointReached -> Navigation.End [order 2] : [NextWaypoint(waypointIndex,route, routeL) == 0]
  StopSimul -> WaitingFlightPlan : after(10,sec)
  (default) -> WaitingFlightPlan
  TakeOff.End -> Navigation
  WaitingFlightPlan -> FlightPlanReceived : [newFP == 1]
  FlightPlanReceived -> TakeOff : [GClock > fp.Dtto]
  Navigation.End -> Landing
  data: moreWaypoint function_output; index function_input; route function_input; routeL function_input; X function_input; d3D function_output; Y function_input; Z function_input; id function_input; cmd output Bus: bus_command; imu input; GClock input; newFP input; fpi input; fpip output; fp local Bus: SL_Bus_autonomous_drone_siam_main_FlightPlan; stop output; posInit local; route local Bus: SL_Bus_autonomous_drone_geometry_msgs_Point; waypointIndex local; routeL local
  function moreWaypoint = NextWaypoint(index, route, routeL):
    | function moreWaypoint = NextWaypoint(index, route, routeL)
    |     if (routeL+1) == index
    |         moreWaypoint = 0;
    |     else
    |         moreWaypoint = 1;
    |     end
    | end
  function d3D = Fly2(X,Y,Z):
    | function d3D = Fly2(X,Y,Z)
    | 
    | fprintf("Volando a %f, %f, %f \n", X, Y ,Z);
    | 
    | % target distance decomposed into earth axes
    | %vector between the commanded position and the drone position
    | dxe = X - imu.posX;
    | dye = Y - imu.posY;
    | dze = Z - imu.posZ;
    | 
    | % target distance
    | % vector3D modulus
    | d3D = norm([dxe;dye;dze]);
    | 
    | % target distance on the plane
    | %vector2D modulus
    | d2D = norm([dxe;dye]);
    | 
    | % angle between drone heading and target
    | %As commanded velocity is relative to drone heading, 
    | %difference between heading and target must be computed in order to compute
    | %the correct drone displacement
    | bearing = atan2d(dye, dxe) - imu.rumbo;
    | 
    | % target distance decomposed into drone body axes
    | %distance transformed to drone taking into account drone heading
    | dx = d2D * cosd(bearing);
    | dy = d2D * sind(bearing);
    | dz = dze;
    | 
    | % velocity obtained from distance
    | % speed softened (50%)
    | vel = [dx;dy;dz]/2;
    | % speed normalization
    | if norm(vel) > 1 
    |     vel = vel / norm(vel);
    | end
    | 
    | fprintf("Volando a %f, %f, %f. Distance: %f \n", X, Y, Z, d3D);
    | 
    | %Speeed commanded
    | cmd.velX = vel(1);
    | cmd.velY = vel(2);
    | cmd.velZ = vel(3);
  function Hover:
    | function Hover
    | 
    | %Keep the drone in the air without displacement
    | cmd.on   = true;
    | cmd.velX = 0;
    | cmd.velY = 0;
    | cmd.velZ = 0;
    | cmd.rotZ = 0;
  function Look2Frame(id):
    | function Look2Frame(id)
    | 
    | %Selection of the frame to look at
    | switch id
    |     case 'red'
    |         fr = cam.red;
    |     case 'green'
    |         fr = cam.green;
    |     case 'blue'
    |         fr = cam.blue;
    | end
    | 
    | %Get the displacement necesary to be in the middle of the frame
    | if (fr.d ~= inf)
    |     HorCenter = (fr.e + fr.w)/2;
    |     cmd.rotZ  = - HorCenter/80;
    |     VerCenter = (fr.n + fr.s)/2;
    |     cmd.velZ  = VerCenter/120;
    | end

== matlab function autonomous_drone/drone simulator/camera bus/ROS communication/vision ==
  data: message input; cam output Bus: bus_camera
function cam = fcn(message)

% leemos la imagen
width  = message.Width;
height = message.Height;
img    = message.Data;

% establecemos los valores umbrales de deteccion de color
th1 = 50;         % umbral entre color primario y secundarios
th2 = 20;         % umbral entre colores secundarios

% marco rojo
frame_red.d = +inf;        % distancia estimada
frame_red.a = +inf;        % angulo de entrada estimado
frame_red.n = +inf;        % lado norte
frame_red.s = -inf;        % lado sur
frame_red.e = -inf;        % lado este
frame_red.w = +inf;        % lado oeste

% marco verde
frame_green = frame_red;      
% marco azul
frame_blue = frame_red; 


% deteccion de rectangulos conteniendo los pixeles de cada marco
i = 1;
for row = 1:height %240
for col = 1:width  %320

    r = double(img(i));  i=i+1;
    g = double(img(i));  i=i+1;
    b = double(img(i));  i=i+1;
    
    if(abs(g-b) < th2) && ((r-g) > th1)        %rojo
        if(frame_red.n > row) 
           frame_red.n = double(row);
        end
        if(frame_red.s < row) 
           frame_red.s = double(row);
        end
        if(frame_red.e < col) 
           frame_red.e = double(col);
        end
        if(frame_red.w > col) 
           frame_red.w = double(col);
        end
    elseif(abs(b-r) < th2) && ((g-b) > th1)    %verde
        if(frame_green.n > row) 
           frame_green.n = double(row);
        end
        if(frame_green.s < row) 
           frame_green.s = double(row);
        end
        if(frame_green.e < col) 
           frame_green.e = double(col);
        end
        if(frame_green.w > col) 
           frame_green.w = double(col);
        end
    elseif(abs(r-g) < th2) && ((b-r) > th1)    %azul
        if(frame_blue.n > row) 
           frame_blue.n = double(row);
        end
        if(frame_blue.s < row) 
           frame_blue.s = double(row);
        end
        if(frame_blue.e < col) 
           frame_blue.e = double(col);
        end
        if(frame_blue.w > col) 
           frame_blue.w = double(col);
        end
    end
    
end
end

% Cambio del sistema de coordenadas de la imagen
frame_red.n   = 120 - frame_red.n;
frame_red.s   = 120 - frame_red.s;
frame_red.e   = frame_red.e - 161;
frame_red.w   = frame_red.w - 161;

frame_green.n = 120 - frame_green.n;
frame_green.s = 120 - frame_green.s;
frame_green.e = frame_green.e - 161;
frame_green.w = frame_green.w - 161;

frame_blue.n  = 120 - frame_blue.n;
frame_blue.s  = 120 - frame_blue.s;
frame_blue.e  = frame_blue.e - 161;
frame_blue.w  = frame_blue.w - 161;


%% Analisis de posicion (distancia, y angulos de deriva/entrada)

d2 = 160^2;    % 160^2 pixeles
L  = 0.23;       % alto de marco
A  = 0.43;       % ancho del marco

if frame_red.n > -inf && frame_red.n < 119 && frame_red.s > -120
    l = frame_red.n - frame_red.s;
    h = frame_red.s + l/2;
    frame_red.d = L/l * sqrt(d2 + h^2);
    ap = frame_red.e - frame_red.w;
    a = max(A/L * l,ap);
    frame_red.a = acosd(ap/a);
end

if frame_green.n > -inf && frame_green.n < 119 && frame_green.s > -120
    l = frame_green.n - frame_green.s;
    h = frame_green.s + l/2;
    frame_green.d = L/l * sqrt(d2 + h^2);
    ap = frame_green.e - frame_green.w;
    a = max(A/L * l,ap);
    frame_green.a = acosd(ap/a);
end

if frame_blue.n > -inf && frame_blue.n < 119 && frame_blue.s > -120
    l = frame_blue.n - frame_blue.s;
    h = frame_blue.s + l/2;
    frame_blue.d = L/l * sqrt(d2 + h^2);
    ap = frame_blue.e - frame_blue.w;
    a = max(A/L * l,ap);
    frame_blue.a = acosd(ap/a);
end




%% Enviamos informacion por el topic
cam.red = frame_red;
cam.green = frame_green;
cam.blue = frame_blue;

== matlab function autonomous_drone/drone simulator/real time control/real time scheduler ==
  data: t_sim input; t_real output
function t_real = fcn(t_sim)
%#codegen

coder.extrinsic('tic');
coder.extrinsic('toc');

persistent t0;
if isempty(t0)
    t0 = tic;
    t_real = 0;
end

t_real = toc(t0);

t_dif = t_sim - t_real;
if t_dif > 0
%    disp(t_dif)
    pause(t_dif);
end

t_real = toc(t0);
%disp(t_real)
